simulink model "KF_AHRS_Dati_Veri"  (R2020b)
settings: Solver=FixedStepAuto  StartTime=0.0  StopTime=T(end)  FixedStep=1/200  RelTol=1e-3
values from neighbouring files (symbols this model uses):
  b_x_vero = -0.3    [init_dati_veri.m]
  b_y_vero = 0.76    [init_dati_veri.m]
  b_z_vero = 0.47    [init_dati_veri.m]
  BARO_cov = single(1.7)/2    [init_1gdl.m]    (also in init_3_gdl_AHRS_fb.m = single(1.7)/5; init_3gdl.m; init_dati_veri.m = single(1.7)/5)
  BARO_cov_old = single(1.7)/2    [init_1gdl.m]    (also in init_3_gdl_AHRS_fb.m; init_3gdl.m; init_dati_veri.m)
  GPS_cov = single([1*2, 1])/2    [init_1gdl.m]    (also in init_3_gdl_AHRS_fb.m = single([0.1*50, 0.1*50, 200*5, 200*5, 0.36])/2; init_3gdl.m = single([1*2, 1*2, 1, 1, 0.36])/2; init_dati_veri.m = single([0.1, 0.1, 200*5, 200*5, 0.36])/2)
  GPS_cov_old = single([0.1, 0.1, 200, 200, 0.36])/2    [init_1gdl.m]    (also in init_3_gdl_AHRS_fb.m = single([0.1, 0.1, 200, 200, 0.36]/2); init_3gdl.m; init_dati_veri.m = single([0.1, 0.1, 200, 200, 0.36]/2))
  IMU_cov = single(15*0.07)/2    [init_1gdl.m]    (also in init_3_gdl_AHRS_fb.m = single([15*[0.07*50, 0.07*50] 15*50*0.09])/2; init_3gdl.m = single([15*[0.07, 0.07] 10*0.09])/2; init_dati_veri.m = single([15*[0.07*5, 0.07*5] 15*50*0.09])/2)
  IMU_cov_old = single([15*[0.07, 0.07] 10*0.09])/2    [init_1gdl.m]    (also in init_3_gdl_AHRS_fb.m = single([15*[0.07, 0.07] 10*0.09]/2); init_3gdl.m; init_dati_veri.m = single([15*[0.07, 0.07] 10*0.09]/2))
  Q = single(diag([1e-2, 1e-6, 1e-4, 1e-12]))*2    [init_1gdl.m]    (also in init_3_gdl_AHRS_fb.m = single(diag([px,vx,ax,py,vy,ay,pz,vz,az,bx,by,bz]))*2; init_3gdl.m = single(diag([px,vx,ax,py,vy,ay,pz,vz,az,bx,by,bz]))*2; init_dati_veri.m = single(diag([px,vx,ax,py,vy,ay,pz,vz,az,bx,by,bz]))*2)
  Q_old = single(diag([1e-8, 1e-1, 1e-2, 1e-8, 1e-1, 1e-2, 1e-5, 1e-4, 0.010]))*2    [init_1gdl.m]    (also in init_3_gdl_AHRS_fb.m; init_3gdl.m; init_dati_veri.m)
  ST = 1/200    (= 0.005)    [init_1gdl.m]    (also in init_3_gdl_AHRS_fb.m; init_3gdl.m; init_dati_veri.m)
  T_50 = 1/50    (= 0.02)    [init_1gdl.m]    (also in init_3_gdl_AHRS_fb.m; init_3gdl.m; init_dati_veri.m)
undefined symbols (not defined in the file or in its folder): DiscIntNeverNeededParam
libraries: simulink x24
(part 3 of 3)

== matlab function KF_AHRS_Dati_Veri/Navigation Filter SINGLE 50 Hz1 ==
  data: flagINITOK input single size=1; flagGPS input single size=1; flagBARO input single size=1; xout output single size=9; measure input single size=9; Q parameter single size=[9,9]; GPS_cov parameter single size=5; BARO_cov parameter single size=1; IMU_cov parameter single size=3; Pout output single
function [xout,Pout] = GPS_BARO_KF_opt( flagINITOK, flagGPS, flagBARO, measure, Q, GPS_cov, BARO_cov, IMU_cov)
%% definition of variables
persistent P %covariance matrix 
persistent x %state vector
persistent filter_running
%filter matrices and constants
persistent A B 
persistent C_GPS_tot R_GPS_tot C_GPS_pos_vel R_GPS_pos_vel C_BARO R_BARO C_IMU R_IMU

if isempty(P)
    P = single(0.1)*Q;
    %initialize state with first measure
    x = single(zeros(9,1));
    
    filter_running = logical(false); %filter starts in OFF, must wait for flagINITOK to become true
    %prepare constant matrices for future use
    dt = single(0.02); 
    %u  = 0;
    subM = [1, dt, 0.5*dt^2;
            0,  1,       dt;
            0,  0,        1];
    A = [subM,zeros(3,3),zeros(3,3);
         zeros(3,3), subM, zeros(3,3);
         zeros(3,3),zeros(3,3),subM];
    B = single(zeros(9,1));
    B(9) = 1; % TODO_:capire che senso ha .... se u= 0 sempre 

    % Covariance state matrix
    % px|vx|ax|py|vy|ay|pz|vz|az
    % Q from mask 

    % Covariance output matrix
    % GPS covariances = px|py|vx|vy|vz
    % GPS_cov  = [0.03, 0.05, 0.016, 0.014, 0.36]; from mask
    % IMU covariances = ax|ay|az
    %IMU_cov  = 1000*[0.07, 0.07, 0.09];    from amsk
    %BARO_cov =  1.7; from amsk 

    %output matrices 
    %tutte le misure disponibili 
    C_GPS_tot = single([ 1 0 0  0 0 0  0 0 0;
                         0 1 0  0 0 0  0 0 0;
                         0 0 1  0 0 0  0 0 0;
                         0 0 0  1 0 0  0 0 0;
                         0 0 0  0 1 0  0 0 0;
                         0 0 0  0 0 1  0 0 0;
                         0 0 0  0 0 0  1 0 0;
                         0 0 0  0 0 0  0 0 1]);
    R_GPS_tot = diag([GPS_cov(1),GPS_cov(3), IMU_cov(1),...
                      GPS_cov(2),GPS_cov(4), IMU_cov(2),...
                      BARO_cov,   IMU_cov(3)]);
    
    % vel GPS, pos GPS & IMU
    C_GPS_pos_vel = single([ 1 0 0  0 0 0  0 0 0;
                             0 1 0  0 0 0  0 0 0;
                             0 0 1  0 0 0  0 0 0;
                             0 0 0  1 0 0  0 0 0;
                             0 0 0  0 1 0  0 0 0;
                             0 0 0  0 0 1  0 0 0;
                             0 0 0  0 0 0  0 0 1]);
                         
    R_GPS_pos_vel = diag([GPS_cov(1),GPS_cov(3), IMU_cov(1),...
                          GPS_cov(2),GPS_cov(4), IMU_cov(2),...
                          IMU_cov(3)]);
    % Baro & IMU
    C_BARO = single([0, 0, 1, 0, 0, 0, 0, 0, 0;
                     0, 0, 0, 0, 0, 1, 0, 0, 0;
                     0, 0, 0, 0, 0, 0, 1, 0, 0         % MANCA ; ????
                     0, 0, 0, 0, 0, 0, 0, 0, 1]);
                 
    R_BARO = diag([IMU_cov(1),...
                   IMU_cov(2),...
                   BARO_cov, IMU_cov(3)]);
    % solo IMU
    C_IMU = single([0, 0, 1, 0, 0, 0, 0, 0, 0;
                    0, 0, 0, 0, 0, 1, 0, 0, 0;
                    0, 0, 0, 0, 0, 0, 0, 0, 1]);
                
    R_IMU = diag([IMU_cov(1),...
                  IMU_cov(2),...
                  IMU_cov(3)]);
    
end

%% initialization 
if and(not(filter_running),flagINITOK),
    % if filter is not running and initialization can be performed 
    % => initialize state = measure
    % => notify filter is running
    x= measure;
    filter_running = true;
end


%% TODO: capire che senso ha mettere u = 0 sempre 
u  = single(0);


if filter_running, 
    %% select update type (removed fuse types with separate gps pos and vel flags)
    if(flagGPS && flagBARO)
        fuse = 1;
    elseif(flagGPS)
        fuse = 2;
    elseif(flagBARO)
        fuse = 7;
    else
        fuse = 8;
    end

    %% Prediction
    [x, P] = predict(A, B, x, u, Q, P);


    %% Update
    switch fuse
        case 1
            % all measurements
            y = [measure(1), measure(2), measure(3), measure(4), measure(5), ...
                 measure(6), measure(7), measure(9)]';
            [x, P] = update(A, C_GPS_tot, x, y, P, R_GPS_tot);
        case 2
            % measurements of: pos GPS, vel GPS, IMU
            y = [measure(1), measure(2), measure(3), measure(4), measure(5), ...
                 measure(6),  measure(9)]';
            [x, P] = update(A, C_GPS_pos_vel, x, y, P, R_GPS_pos_vel);
        case 7
            % measurements of: BARO, IMU
            y = [measure(3), measure(6), measure(7), measure(9)]';
            [x, P] = update(A, C_BARO, x, y, P, R_BARO);
        case 8
            y = [measure(3), measure(6), measure(9)]';
            [x, P] = update(A, C_IMU, x, y, P, R_IMU);
    end
end

xout = x;
Pout = P;
end

function [x, P] = predict(A, B, x, u, Q, P)
    x = A*x + B*u;
    P = A*P*A' + Q;
end

function [x, P] = update(A, C, x, y, P, R)
    K = P*C'*inv(R + C*P*C');
    x = x + K*(y - C*x);
    P = (eye(9) - K*C)*P;
    %P = 0.5*(P + transpose(P)); secondo me ci va, non dovrebbe fare male
end

== matlab function KF_AHRS_Dati_Veri/MPU AHRS1/Attitude Filter MPU/DCM_MARG_QUAT/dcm_marg ==
  data: euler_out output single; a_ned output single; gyro input single; acc input single; mag input single; q input single; e_int_a input single; e_int_m input single; q_out output single; Kp parameter single; Ki parameter single; T parameter single; e_int_out_a output single; e_int_out_m output single; Rt output; biases output single
function [euler_out, a_ned, q_out, e_int_out_a, e_int_out_m,Rt, biases] = fcn(gyro, acc, mag, q, e_int_a, e_int_m, Kp, Ki, T)
%#codegen

persistent ini;

% mode == 0: magnetos' errors don't affect roll and pitch angles
% mode == 1: standard implementation, roll, pitch and yaw depend on
% acceleroters and magnetos in the same measure
mode = 0;

% Magnetos and accelerometers MUST have non null norm, if they have null
% norm an error occurred and filter probably will get confused, adjust mag
% and acc values to try to avoid filter problems. 

if (norm(acc) < 1e-4)
    acc = single([0; 0; -9.81]);
end

if (norm(mag) < 1e-4)
    mag = single([0.234; 0.008; 0.404]);
end

% Init quaternion using the first accelerometers and magnetometers reading
% in triad algorithm.

if (isempty(ini))
    q = qtriad(acc, mag);
    ini = 1;
end

q1 = q(1);
q2 = q(2);
q3 = q(3);
q4 = q(4);

gx = gyro(1);
gy = gyro(2);
gz = gyro(3);

ax = acc(1);
ay = acc(2);
az = acc(3);

mx = mag(1);
my = mag(2);
mz = mag(3);

% Rt rotates NED to body, and obviously converts body cordinates into ned
% coordinates.
 
Rt = [1 - 2*q3^2 - 2*q4^2, 2*(q2*q3-q1*q4), 2*(q2*q4+q1*q3);
      2*(q2*q3+q1*q4), 1 - 2*q2^2 - 2*q4^2, 2*(q3*q4-q1*q2);
      2*(q2*q4-q1*q3), 2*(q3*q4+q1*q2), 1 - 2*q2^2 - 2*q3^2];

% Filter implementation, see article for details
 
h = Rt*[mx; my; mz];

bx = sqrt(h(1)^2+h(2)^2);
bz = abs(h(3));

norm_a = sqrt(ax^2+ay^2+az^2+eps);
e_a = cross([ax ay az]'/norm_a, Rt'*[0 0 -1]');
norm_m = sqrt(mx^2+my^2+mz^2+eps);
norm_b = sqrt(bx^2+bz^2+eps);
e_m = cross([mx my mz]'/norm_m, Rt'*[bx 0 bz]'/norm_b);
% e_m = single(zeros(3,1)); %no mag correction
if (mode == 0)
    
    e_int_out_a = e_int_a + T*[e_a(1:2); 0];
    e_int_out_m = e_int_m + T*[0; 0; e_m(3)];
%     e_int_out_m = single(zeros(3,1)); 
    g = [gx; gy; gz] + Kp*[e_a(1:2); e_m(3)] + Ki*(e_int_out_a + e_int_out_m);

else
    
    e_int_out_a = e_int_a + T*e_a;
    e_int_out_m = e_int_m + T*e_m;
%     e_int_out_m = single(zeros(3,1));
    g = [gx; gy; gz] + Kp*(e_a + e_m) + Ki*(e_int_out_a + e_int_out_m);
    
end

gx = g(1);
gy = g(2);
gz = g(3);

% Quaternion integration

dq1 = (-q2*gx - q3*gy - q4*gz)/2;
dq2 = (q1*gx + q3*gz - q4*gy)/2;
dq3 = (q1*gy - q2*gz + q4*gx)/2;
dq4 = (q1*gz + q2*gy - q3*gx)/2;

q1 = q1 + dq1*T;
q2 = q2 + dq2*T;
q3 = q3 + dq3*T;
q4 = q4 + dq4*T;

% Quaternion normalization

norm_q = sqrt(q1*q1 + q2*q2 + q3*q3 + q4*q4);
q1 = q1 / norm_q;
q2 = q2 / norm_q;
q3 = q3 / norm_q;
q4 = q4 / norm_q;

q_out = [q1; q2; q3; q4];

% Rt rotates NED to body, and obviously converts body cordinates into ned
% coordinates.

Rt = [1 - 2*q3^2 - 2*q4^2, 2*(q2*q3-q1*q4), 2*(q2*q4+q1*q3);
      2*(q2*q3+q1*q4), 1 - 2*q2^2 - 2*q4^2, 2*(q3*q4-q1*q2);
      2*(q2*q4-q1*q3), 2*(q3*q4+q1*q2), 1 - 2*q2^2 - 2*q3^2];

% Obtain rpy angles
 
psi = atan2(2*(q2*q3+q1*q4), 1 - 2*q3^2 - 2*q4^2);
theta = atan2(-2*(q2*q4-q1*q3), sqrt((2*(q3*q4+q1*q2))^2 + (1 - 2*q2^2 - 2*q3^2)^2));
phi = atan2(2*(q3*q4+q1*q2), 1 - 2*q2^2 - 2*q3^2);

% Compute accelerations in NED

a_ned = Rt*acc;

euler_out = [phi; theta; psi];

% Suppose that mean of integral correction is bias value

biases = -Ki*(e_int_out_a + e_int_out_m);

end

function R = rotz(a)
R = [ cos(a), -sin(a), 0; sin(a), cos(a), 0 ; 0, 0, 1];
end

function R = rotx(a)
R = [ 1, 0, 0; 0, cos(a), -sin(a); 0, sin(a), cos(a);];
end

function R = roty(a)
R = [ cos(a), 0, sin(a) ; 0, 1, 0, ; -sin(a), 0, cos(a)];
end

% Triad algorithm

function q_out = qtriad(acc, mag)

ib = acc/norm(acc);
ir = [0; 0; -1];
mb = mag;
mr = [0.234; 0.008; 0.404];
jb = cross(ib,mb);
jb = jb/norm(jb);
jr = cross(ir,mr);
jr = jr/norm(jr);
kb = cross(ib,jb);
kr = cross(ir,jr);
c = (ib*ir' + jb*jr' + kb*kr')';

q1 = 0.5*sqrt(1+c(1,1)+c(2,2)+c(3,3));
q2 = 0.25/q1*(c(3,2)-c(2,3));
q3 = 0.25/q1*(c(1,3)-c(3,1));
q4 = 0.25/q1*(c(2,1)-c(1,2));

q_out = [q1 q2 q3 q4]';
    
end
